simulink model "sample2_realistic_diapason"  (R2014a)
settings: Solver=ode45  StartTime=0.0  StopTime=10.0  RelTol=1e-3
settings Model: Creator=simoz  LastModifiedBy=simoz

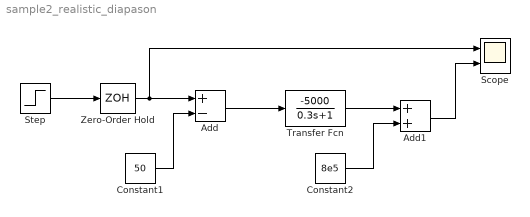
== system sample2_realistic_diapason ==
  Add : Sum  Inputs=+-
  Add1 : Sum
  Constant1 : Constant  Value=50
  Constant2 : Constant  Value=8e5
  Scope : Scope  NumInputPorts=2
      settings: YMin=-5~-5  YMax=5~5
  Step : Step  Before=50  After=60  SampleTime=0
  Transfer Fcn : TransferFcn  Numerator=[-5000]  Denominator=[0.3 1]
  Zero-Order Hold : ZeroOrderHold  SampleTime=0.5
  wires:
  Zero-Order Hold/1 -> Add/1, Scope/1
  Add/1 -> Transfer Fcn/1
  Constant1/1 -> Add/2
  Transfer Fcn/1 -> Add1/1
  Add1/1 -> Scope/2
  Constant2/1 -> Add1/2
  Step/1 -> Zero-Order Hold/1
